simulink model "model"  (R2020b)
settings: Solver=VariableStepAuto  StartTime=0.0  StopTime=1800  RelTol=1e-3
PostLoadFcn:
  | cd(fileparts(which(bdroot)));
  | close all;
  | clear all;
  | clc;
  | set_param('model/switch_v','Label','');
  | set_param('model/switch_h','Label','');
  | set_param('model/switch_T','Label','');
  | set_param('model/switch_P','Label','');
  | set_param('model/switch_m','Label','');
  | set_param('model/switch_p','Label','');
  | set_param('model/switch_slope','Label','');
  | set_param('model/pEtrac','ShowInitialText','off');
  | set_param('model/pErreur+','ShowInitialText','off');
  | set_param('model/pErreur-','ShowInitialText','off');
  | set_param('model/Emodel/Etrac et Erreur/pEtrac','Value','0');
  | set_param('model/Emodel/Etrac et Erreur/pErreur+','Value','0');
  | set_param('model/Emodel/Etrac et Erreur/pErreur-','Value','0');
InitFcn:
  | cd(fileparts(which(bdroot)));
  | load('cycles.mat');
  | clear cycles;
  | cycles = who('-file','cycles.mat');
  | cycleNum = str2num(get_param('model/Emodel/switch_cycles','Value'));
  | cycleName = char(cycles(cycleNum));
  | set_param('model/Emodel/cycle','VariableName',cycleName);
  | cycle = evalin('base',cycleName);
  | T = cycle.time(end);
  | cycleLength = string(T);
  | set_param('model','StopTime',cycleLength);
  | 
  | try
  |  pEtrac = get_param('model/Etrac','Value');
  |  pEtrac = split(pEtrac,'"');
  |  pEtrac = string(pEtrac(2));
  |  set_param('model/Emodel/Etrac et Erreur/pEtrac','Value',pEtrac);
  | 
  |  pErreup = get_param('model/Erreur+','Value');
  |  pErreup = split(pErreup,'"');
  |  pErreup = string(pErreup(2));
  |  set_param('model/Emodel/Etrac et Erreur/pErreur+','Value',pErreup);
  | 
  |  pErreum = get_param('model/Erreur-','Value');
  |  pErreum = split(pErreum,'"');
  |  pErreum = string(pErreum(2));
  |  set_param('model/Emodel/Etrac et Erreur/pErreur-','Value',pErreum);
  | end
StopFcn:
  | sig1Colors.Color = [0 0 1];
  | sig1Colors.LineStyle = '-';
  | sig2Colors.Color = [1 0 0];
  | sig2Colors.LineStyle = '-';
  | sig3Colors.Color = [1 0 0];
  | sig3Colors.LineStyle = '-';
  | sigColors = [sig1Colors sig2Colors sig3Colors];
  | set_param('model/Dashboard_Etrac','Colors',sigColors);
libraries: simulink x1
settings Model: PacingRate=1000  Creator=calexandre  LastModifiedBy=calexandre

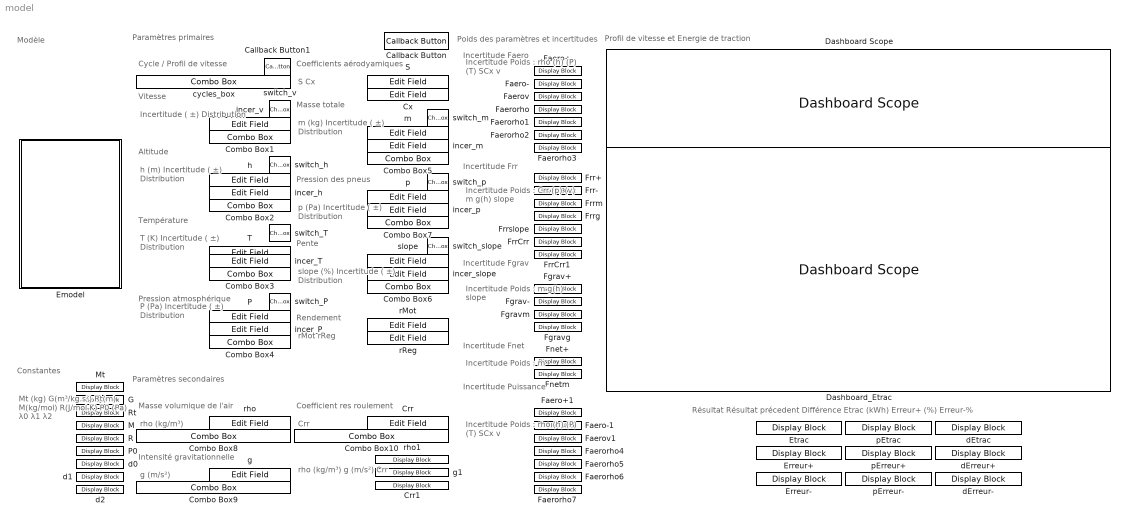
== system model ==
  note: Mt (kg)
      | G(m³/kg.s²)
      | Rt(m)
      | M(kg/mol)
      | R(J/mol.K)
      | P0 (Pa)
      | λ0
      | λ1
      | λ2
  note: Résultat
      | Résultat précedent
      | Différence
      |
      | Etrac (kWh)
      |
      | Erreur+ (%)
      |
      | Erreur-%
  note: Profil de vitesse et Energie de traction
  note: Modèle
  note: Paramètres primaires
  note: Cycle / Profil de vitesse
  note: Incertitude ( ±)
      | Distribution
  note: h (m)
      | Incertitude ( ±)
      | Distribution
  note: Altitude
  note: T (K)
      | Incertitude ( ±)
      | Distribution
  note: Température
  note: P (Pa)
      | Incertitude ( ±)
      | Distribution
  note: Pression atmosphérique
  note: m (kg)
      | Incertitude ( ±)
      | Distribution
  note: Masse totale
  note: slope (%)
      | Incertitude ( ±)
      | Distribution
  note: Pente
  note: p (Pa)
      | Incertitude ( ±)
      | Distribution
  note: Pression des pneus
  note: rho (kg/m³)
  note: Masse volumique de l'air
  note: g (m/s²)
  note: Intensité gravitationnelle
  note: Crr
  note: Coefficient res roulement
  note: S
      | Cx
  note: Coefficients aérodyamiques
  note: Rendement
  note: rMot
      | rReg
  note: Paramètres secondaires
  note: Vitesse
  note: Constantes
  note: Poids des paramètres et incertitudes
  note: rho (kg/m³)
      | g (m/s²)
      | Crr
  note: Incertitude
      | Poids : rho
      | (h)
      | (P)
      | (T)
      | SCx
      | v
  note: Incertitude Faero
  note: Incertitude
      | Poids : Crr
      | (p)
      | (v)
      | m
      | g(h)
      | slope
  note: Incertitude Frr
  note: Incertitude Fgrav
  note: Incertitude
      | Poids : m
      | g(h)
      | slope
  note: Incertitude Fnet
  note: Incertitude
      | Poids : m
  note: Incertitude
      | Poids : rho
      | (h)
      | (P)
      | (T)
      | SCx
      | v
  note: Incertitude Puissance
  Callback Button : CallbackButton  ButtonText=Reset
      settings: ClickFcn=|
      | set_param('model/Emodel/h(m)','Value','0');
      | set_param('model/Emodel/T(K)','Value','285');
      | set_param('model/Emodel/P(Pa)','Value','102900');
      | set_param('model/Emodel/S','Value','2.3');
      | set_param('model/Emodel/Cx','Value','0.36');
      | set_param('model/Emodel/m(kg)','Value','1240');
      | set_param('model/Emodel/p(Pa)','Value','200000');
      | set_param('model/Emodel/slope(%)','Value','0');
      | set_param('model/Emodel/rho(kg.m-3)','Value','1.292');
      | set_param('model/Emodel/g(m.s-2)','Value','9.81');
      | 
      | set_param('model/Emodel/incertitude v','Value','0');
      | set_param('model/Emodel/incertitude h','Value','0');
      | set_param('model/Emodel/incertitude T','Value','0');
      | set_param('model/Emodel/incertitude P','Value','0');
      | set_param('model/Emodel/incertitude m','Value','0');
      | set_param('model/Emodel/incertitude p','Value','0');
      | set_param('model/Emodel/incertitude slope','Value','0');
      | 
      | set_param('model/Emodel/switch incertitude v','Value','0');
      | set_param('model/Emodel/switch incertitude h','Value','0');
      | set_param('model/Emodel/switch incertitude T','Value','0');
      | set_param('model/Emodel/switch incertitude P','Value','0');
      | set_param('model/Emodel/switch incertitude m','Value','0');
      | set_param('model/Emodel/switch incertitude p','Value','0');
      | set_param('model/Emodel/switch incertitude slope','Value','0');
      | 
      | set_param('model/h','FontSize','11');
      | set_param('model/T','FontSize','11');
      | set_param('model/P','FontSize','11');
      | set_param('model/S','FontSize','11');
      | set_param('model/Cx','FontSize','11');
      | set_param('model/m','FontSize','11');
      | set_param('model/p','FontSize','11');
      | set_param('model/slope','FontSize','11');
      | set_param('model/rMot','FontSize','11');
      | set_param('model/rReg','FontSize','11');
      | set_param('model/rho','FontSize','11');
      | set_param('model/g','FontSize','11');
      | set_param('model/Crr','FontSize','11');
      | set_param('model/incer_v','FontSize','11');
      | set_param('model/incer_h','FontSize','11');
      | set_param('model/incer_T','FontSize','11');
      | set_param('model/incer_P','FontSize','11');
      | set_param('model/incer_m','FontSize','11');
      | set_param('model/incer_p','FontSize','11');
      | set_param('model/incer_slope','FontSize','11');
      | set_param('model/Mt','FontSize','11');
      | set_param('model/G','FontSize','11');
      | set_param('model/Rt','FontSize','11');
      | set_param('model/M','FontSize','11');
      | set_param('model/R','FontSize','11');
      | set_param('model/P0','FontSize','11');
      | set_param('model/d0','FontSize','11');
      | set_param('model/d1','FontSize','11');
      | set_param('model/d2','FontSize','11');
      | set_param('model/Etrac','FontSize','11');
      | set_param('model/Erreur+','FontSize','11');
      | set_param('model/Erreur-','FontSize','11');
      | set_param('model/pEtrac','FontSize','11');
      | set_param('model/pErreur+','FontSize','11');
      | set_param('model/pErreur-','FontSize','11');
      | set_param('model/dEtrac','FontSize','11');
      | set_param('model/dErreur+','FontSize','11');
      | set_param('model/dErreur-','FontSize','11');
      | set_param('model/rho1','FontSize','11');
      | set_param('model/g1','FontSize','11');
      | set_param('model/Crr1','FontSize','11');
      | 
      | set_param('model/h','FontSize','12');
      | set_param('model/T','FontSize','12');
      | set_param('model/P','FontSize','12');
      | set_param('model/S','FontSize','12');
      | set_param('model/Cx','FontSize','12');
      | set_param('model/m','FontSize','12');
      | set_param('model/p','FontSize','12');
      | set_param('model/slope','FontSize','12');
      | set_param('model/rMot','FontSize','12');
      | set_param('model/rReg','FontSize','12');
      | set_param('model/rho','FontSize','12');
      | set_param('model/g','FontSize','12');
      | set_param('model/Crr','FontSize','12');
      | set_param('model/incer_v','FontSize','12');
      | set_param('model/incer_h','FontSize','12');
      | set_param('model/incer_T','FontSize','12');
      | set_param('model/incer_P','FontSize','12');
      | set_param('model/incer_m','FontSize','12');
      | set_param('model/incer_p','FontSize','12');
      | set_param('model/incer_slope','FontSize','12');
      | set_param('model/Mt','FontSize','12');
      | set_param('model/G','FontSize','12');
      | set_param('model/Rt','FontSize','12');
      | set_param('model/M','FontSize','12');
      | set_param('model/R','FontSize','12');
      | set_param('model/P0','FontSize','12');
      | set_param('model/d0','FontSize','12');
      | set_param('model/d1','FontSize','12');
      | set_param('model/d2','FontSize','12');
      | set_param('model/Etrac','FontSize','16');
      | set_param('model/Erreur+','FontSize','16');
      | set_param('model/Erreur-','FontSize','16');
      | set_param('model/pEtrac','FontSize','16');
      | set_param('model/pErreur+','FontSize','16');
      | set_param('model/pErreur-','FontSize','16');
      | set_param('model/dEtrac','FontSize','16');
      | set_param('model/dErreur+','FontSize','16');
      | set_param('model/dErreur-','FontSize','16');
      | set_param('model/rho1','FontSize','12');
      | set_param('model/g1','FontSize','12');
      | set_param('model/Crr1','FontSize','12');
  Callback Button1 : CallbackButton  ButtonText=↺
      settings: ClickFcn=|
      | cd(fileparts(which(bdroot)));
      | clear cycles;
      | clear cycles_box_states;
      | cycles = who('-file','cycles.mat');
      | cycles_box_states(length(cycles)) = struct();
      | for i = 1:length(cycles)
      | 	cycles_box_states(i).Value = i;
      |     cycles_box_states(i).Label = char(cycles(i));
      | end
      | set_param('model/cycles_box','States',cycles_box_states);
  Combo Box{1..7} (7 alike) : ComboBox  LabelPosition=Hide  SelectedLabel=Incer-type
      settings: Values={{'Incer-type', 'Gaussienne', 'Rectangulaire', 'Triangle', 'Normale', 'en U'}, [1 2 3 4 5 6]}
  Combo Box10 : ComboBox  LabelPosition=Hide  SelectedLabel=Valeur nominale
      settings: Values={{'Valeur nominale', 'f(p,v)'}, [1 0]}
  Combo Box8 : ComboBox  LabelPosition=Hide  SelectedLabel=Valeur nominale
      settings: Values={{'f(P,T)', 'f(h,T)', 'Valeur nominale'}, [1 2 3]}
  Combo Box9 : ComboBox  LabelPosition=Hide  SelectedLabel=Valeur nominale
      settings: Values={{'Valeur nominale', 'f(h)'}, [0 1]}
  Crr : EditField  LabelPosition=Hide  ShowInitialText=on  Alignment=Center
  Crr1 : DisplayBlock  LabelPosition=Hide  Format=Custom  Transparency=1  FormatString=%.4f
  Cx : EditField  LabelPosition=Hide  ShowInitialText=on  Alignment=Center
  Dashboard Scope : DashboardScope
  Dashboard_Etrac : DashboardScope
  Emodel : Subsystem
  Erreur+ : DisplayBlock  LabelPosition=Hide  Format=short  Transparency=1
  Erreur- : DisplayBlock  LabelPosition=Hide  Format=short  Transparency=1
  Etrac : DisplayBlock  LabelPosition=Hide  Format=short  Transparency=1
  Faero+ : DisplayBlock  LabelPosition=Hide  Format=Custom  Alignment=Right  Transparency=1  FormatString=%.2f N
  Faero+1 : DisplayBlock  LabelPosition=Hide  Format=Custom  Alignment=Right  Transparency=1  FormatString=%.2f N
  Faero- : DisplayBlock  LabelPosition=Hide  Format=Custom  Alignment=Right  Transparency=1  FormatString=%.2f N
  Faero-1 : DisplayBlock  LabelPosition=Hide  Format=Custom  Alignment=Right  Transparency=1  FormatString=%.2f N
  Faerorho{,1..7} (8 alike) : DisplayBlock  LabelPosition=Hide  Format=Custom  Alignment=Right  Transparency=1  FormatString=%.1f %%
  Faerov : DisplayBlock  LabelPosition=Hide  Format=Custom  Alignment=Right  Transparency=1  FormatString=%.1f %%
  Faerov1 : DisplayBlock  LabelPosition=Hide  Format=Custom  Alignment=Right  Transparency=1  FormatString=%.1f %%
  Fgrav+ : DisplayBlock  LabelPosition=Hide  Format=Custom  Alignment=Right  Transparency=1  FormatString=%.2f N
  Fgrav- : DisplayBlock  LabelPosition=Hide  Format=Custom  Alignment=Right  Transparency=1  FormatString=%.2f N
  Fgravg : DisplayBlock  LabelPosition=Hide  Format=Custom  Alignment=Right  Transparency=1  FormatString=%.1f %%
  Fgravm : DisplayBlock  LabelPosition=Hide  Format=Custom  Alignment=Right  Transparency=1  FormatString=%.1f %%
  Fnet+ : DisplayBlock  LabelPosition=Hide  Format=Custom  Alignment=Right  Transparency=1  FormatString=%.2f N
  Fnetm : DisplayBlock  LabelPosition=Hide  Format=Custom  Alignment=Right  Transparency=1  FormatString=%.1f %%
  Frr+ : DisplayBlock  LabelPosition=Hide  Format=Custom  Alignment=Right  Transparency=1  FormatString=%.2f N
  Frr- : DisplayBlock  LabelPosition=Hide  Format=Custom  Alignment=Right  Transparency=1  FormatString=%.2f N
  FrrCrr : DisplayBlock  LabelPosition=Hide  Format=Custom  Alignment=Right  Transparency=1  FormatString=%.1f %%
  FrrCrr1 : DisplayBlock  LabelPosition=Hide  Format=Custom  Alignment=Right  Transparency=1  FormatString=%.1f %%
  Frrg : DisplayBlock  LabelPosition=Hide  Format=Custom  Alignment=Right  Transparency=1  FormatString=%.1f %%
  Frrm : DisplayBlock  LabelPosition=Hide  Format=Custom  Alignment=Right  Transparency=1  FormatString=%.1f %%
  Frrslope : DisplayBlock  LabelPosition=Hide  Format=Custom  Alignment=Right  Transparency=1  FormatString=%.1f %%
  G : DisplayBlock  LabelPosition=Hide  Format=short  Transparency=1
  M : DisplayBlock  LabelPosition=Hide  Format=short  Transparency=1
  Mt : DisplayBlock  LabelPosition=Hide  Format=short  Transparency=1
  P : EditField  LabelPosition=Hide  ShowInitialText=on  Alignment=Center
  P0 : DisplayBlock  LabelPosition=Hide  Format=short  Transparency=1
  R : DisplayBlock  LabelPosition=Hide  Format=short  Transparency=1
  Rt : DisplayBlock  LabelPosition=Hide  Format=short  Transparency=1
  S : EditField  LabelPosition=Hide  ShowInitialText=on  Alignment=Center
  T : EditField  LabelPosition=Hide  ShowInitialText=on  Alignment=Center
  cycles_box : ComboBox  LabelPosition=Hide  SelectedLabel=WLTP_class_3
      settings: Values={{'ArtMw130', 'ArtMw150', 'ArtRoad', 'ArtUrban', 'ECE_R15', 'EUDC', 'FTP', 'HWFET', 'NEDC', 'UDDS', 'WLTP', 'WLTP_class_3'}, [1 2 3 4 5 6 7 8 9 10 11 12]}
  d0 : DisplayBlock  LabelPosition=Hide  Format=short  Transparency=1
  d1 : DisplayBlock  LabelPosition=Hide  Format=short  Transparency=1
  d2 : DisplayBlock  LabelPosition=Hide  Format=short  Transparency=1
  dErreur+ : DisplayBlock  LabelPosition=Hide  ShowInitialText=off  Format=short  Transparency=1
  dErreur- : DisplayBlock  LabelPosition=Hide  ShowInitialText=off  Format=short  Transparency=1
  dEtrac : DisplayBlock  LabelPosition=Hide  ShowInitialText=off  Format=short  Transparency=1
  g : EditField  LabelPosition=Hide  ShowInitialText=on  Alignment=Center
  g1 : DisplayBlock  LabelPosition=Hide  Format=Custom  Transparency=1  FormatString=%.3f m/s²
  h : EditField  LabelPosition=Hide  ShowInitialText=on  Alignment=Center
  incer_P : EditField  LabelPosition=Hide  ShowInitialText=on  Alignment=Center
  incer_T : EditField  LabelPosition=Hide  ShowInitialText=on  Alignment=Center
  incer_h : EditField  LabelPosition=Hide  ShowInitialText=on  Alignment=Center
  incer_m : EditField  LabelPosition=Hide  ShowInitialText=on  Alignment=Center
  incer_p : EditField  LabelPosition=Hide  ShowInitialText=on  Alignment=Center
  incer_slope : EditField  LabelPosition=Hide  ShowInitialText=on  Alignment=Center
  incer_v : EditField  LabelPosition=Hide  ShowInitialText=on  Alignment=Center
  m : EditField  LabelPosition=Hide  ShowInitialText=on  Alignment=Center
  p : EditField  LabelPosition=Hide  ShowInitialText=on  Alignment=Center
  pErreur+ : DisplayBlock  LabelPosition=Hide  ShowInitialText=off  Format=short  Transparency=1
  pErreur- : DisplayBlock  LabelPosition=Hide  ShowInitialText=off  Format=short  Transparency=1
  pEtrac : DisplayBlock  LabelPosition=Hide  ShowInitialText=off  Format=short  Transparency=1
  rMot : EditField  LabelPosition=Hide  ShowInitialText=on  Alignment=Center
  rReg : EditField  LabelPosition=Hide  ShowInitialText=on  Alignment=Center
  rho : EditField  LabelPosition=Hide  ShowInitialText=on  Alignment=Center
  rho1 : DisplayBlock  LabelPosition=Hide  Format=Custom  Transparency=1  FormatString=%.3f kg/m³
  slope : EditField  LabelPosition=Hide  ShowInitialText=on  Alignment=Center
  switch_P : Checkbox  LabelPosition=Hide  ShowInitialText=on
  switch_T : Checkbox  LabelPosition=Hide  ShowInitialText=on
  switch_h : Checkbox  LabelPosition=Hide  ShowInitialText=on
  switch_m : Checkbox  LabelPosition=Hide  ShowInitialText=on
  switch_p : Checkbox  LabelPosition=Hide  ShowInitialText=on
  switch_slope : Checkbox  LabelPosition=Hide  ShowInitialText=on
  switch_v : Checkbox  LabelPosition=Hide  ShowInitialText=on

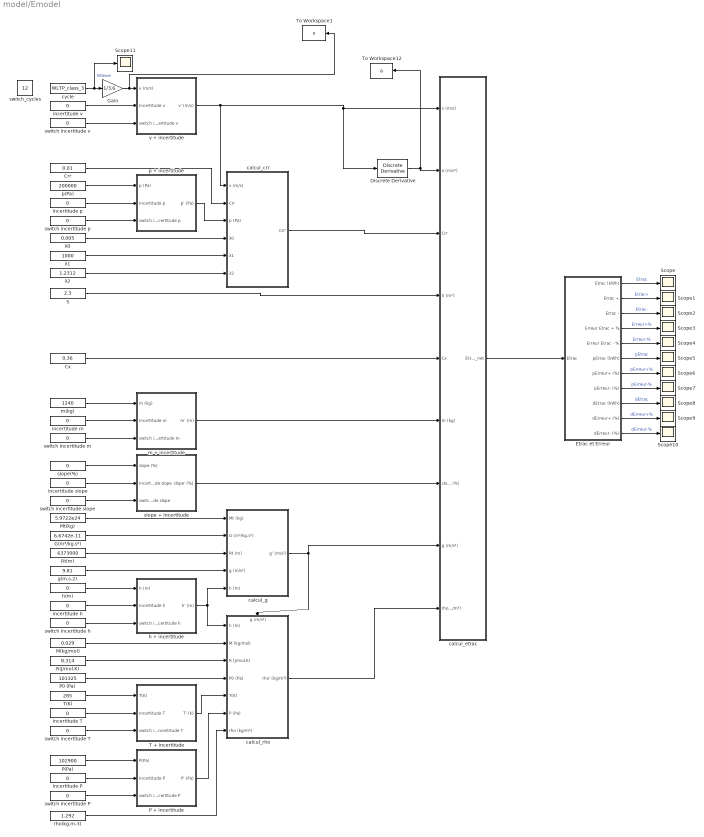
== system model/Emodel ==
  Crr : Constant  Value=0.01
  Cx : Constant  Value=0.36
  Discrete Derivative : simulink/Discrete/Discrete Derivative  gainval=1.0  ICPrevScaledInput=0.0  OutMin=[]  OutMax=[]  OutDataType=fixdt(1, 16)  OutScaling=2^-10  DoSatur=off
  Etrac et Erreur : Subsystem
  G(m³/kg.s²) : Constant  Value=6.6742e-11
  Gain : Gain  Gain=1/3.6
  M(kg/mol) : Constant  Value=0.029
  Mt(kg) : Constant  Value=5.9722e24
  P + incertitude : Subsystem
  P(Pa) : Constant  Value=102900
  P0 (Pa) : Constant  Value=101325
  R(J/mol.K) : Constant  Value=8.314
  Rt(m) : Constant  Value=6373000
  S : Constant  Value=2.3
  Scope{,1..11} (12 alike) : Scope
  T + incertitude : Subsystem
  T(K) : Constant  Value=285
  To Workspace1 : ToWorkspace  VariableName=v  SampleTime=-1
  To Workspace12 : ToWorkspace  VariableName=a  SampleTime=-1
  calcul_crr : Subsystem
  calcul_etrac : Subsystem
  calcul_g : Subsystem
  calcul_rho : Subsystem
      settings: PortSchema="{\"entries\":[{\"content\":{\"sides\":[{\"content\":{\"connectorIds\":[\"In1\",\"In2\",\"In3\",\"In4\",\"In5\",\"In6\",\"In7\"]},\"type\":\"ConnectorPlacement.EquallySpacedRectSide\",\"uuid\":\"cc83d484-c74b-48b3-b83e-1c0f0a113df0\"},{\"content\":{\"connectorIds\":[\"Out1\"],\"side\":\"RIGHT\"},\"type\":\"ConnectorPlacement.EquallySpacedRectSide\",\"uuid\":\"f49ce46b-81e5-420e-b383-21adfa8decb6\"},{\"content\":{\"connectorIds\":[\"In8\"],\"side\":\"TOP\"},\"type\":\"ConnectorPlacement.EquallySpacedRectSide\",\"uuid\":\"3a8f1516-3d8d-4158-a843-5a7993412ec1\"},{\"content\":{\"connectorIds\":[],\"side\":\"HIDDEN\"},\"type\":\"ConnectorPlacement.EquallySpacedRectSide\",\"uuid\":\"5a38b1a2-2dd9-418a-a84f-c8a924db452d\"}]},\"type\":\"ConnectorPlacement.EquallySpacedConnector\",\"uuid\":\"39c01f9e-7b83-41af-a371-ba0a6382fb58\"}],\"packageUris\":[\"http://schema.mathworks.com/mf0/Connector/R2020b\"],\"version\":\"1.0\"}"
  cycle : FromWorkspace  VariableName=WLTP_class_3  SampleTime=1
  g(m.s-2) : Constant  Value=9.81
  h + incertitude : Subsystem
  h(m) : Constant  Value=0
  incertitude P : Constant  Value=0
  incertitude T : Constant  Value=0
  incertitude h : Constant  Value=0
  incertitude m : Constant  Value=0
  incertitude p : Constant  Value=0
  incertitude slope : Constant  Value=0
  incertitude v : Constant  Value=0
  m + incertitude : Subsystem
  m(kg) : Constant  Value=1240
  p + incertitude : Subsystem
  p(Pa) : Constant  Value=200000
  rho(kg.m-3) : Constant  Value=1.292
  slope + incertitude : Subsystem
  slope(%) : Constant  Value=0
  switch incertitude P : Constant  Value=0
  switch incertitude T : Constant  Value=0
  switch incertitude h : Constant  Value=0
  switch incertitude m : Constant  Value=0
  switch incertitude p : Constant  Value=0
  switch incertitude slope : Constant  Value=0
  switch incertitude v : Constant  Value=0
  switch_cycles : Constant  Value=12
  v + incertitude : Subsystem
  λ0 : Constant  Value=0.005
  λ1 : Constant  Value=1000
  λ2 : Constant  Value=1.2312
  wires:
  v + incertitude/1(v' (m/s)) -> calcul_crr/1(v (m/s)), Discrete Derivative/1, calcul_etrac/1(v (m/s))
  Cx/1 -> calcul_etrac/5(Cx)
  S/1 -> calcul_etrac/4(S (m²))
  m + incertitude/1(m' (m)) -> calcul_etrac/6(m (kg))
  M(kg/mol)/1 -> calcul_rho/2(M (kg/mol))
  R(J/mol.K)/1 -> calcul_rho/3(R (J/mol.K))
  calcul_rho/1(rho' (kg/m³)) -> calcul_etrac/9(rho (kg/m³))
  calcul_g/1(g' (m/s²)) -> calcul_rho/8(g (m/s²)), calcul_etrac/8(g (m/s²))
  Mt(kg)/1 -> calcul_g/1(Mt (kg))
  G(m³/kg.s²)/1 -> calcul_g/2(G (m³/kg.s²))
  Rt(m)/1 -> calcul_g/3(Rt (m))
  h + incertitude/1(h' (m)) -> calcul_rho/1(h (m)), calcul_g/5(h (m))
  h(m)/1 -> h + incertitude/1(h (m))
  incertitude h/1 -> h + incertitude/2(Incertitude h)
  switch incertitude h/1 -> h + incertitude/3(switch incertitude h)
  calcul_crr/1(Crr') -> calcul_etrac/3(Crr)
  p(Pa)/1 -> p + incertitude/1(p (Pa))
  p + incertitude/1(p' (Pa)) -> calcul_crr/3(p (Pa))
  incertitude p/1 -> p + incertitude/2(Incertitude p)
  T(K)/1 -> T + incertitude/1(T(K))
  T + incertitude/1(T' (k)) -> calcul_rho/5(T(K))
  switch incertitude T/1 -> T + incertitude/3(switch incertitude T)
  incertitude T/1 -> T + incertitude/2(Incertitude T)
  switch incertitude p/1 -> p + incertitude/3(switch incertitude p)
  switch incertitude slope/1 -> slope + incertitude/3(switch incertitude slope)
  incertitude slope/1 -> slope + incertitude/2(Incertitude slope)
  slope(%)/1 -> slope + incertitude/1(slope (%))
  switch incertitude m/1 -> m + incertitude/3(switch incertitude m)
  incertitude m/1 -> m + incertitude/2(Incertitude m)
  m(kg)/1 -> m + incertitude/1(m (kg))
  slope + incertitude/1(slope' (%)) -> calcul_etrac/7(slope (%))
  Gain/1 -> To Workspace1/1, v + incertitude/1(v (m/s))
  incertitude v/1 -> v + incertitude/2(Incertitude v)
  switch incertitude v/1 -> v + incertitude/3(switch incertitude v)
  P(Pa)/1 -> P + incertitude/1(P(Pa))
  incertitude P/1 -> P + incertitude/2(Incertitude P)
  switch incertitude P/1 -> P + incertitude/3(switch incertitude P)
  P + incertitude/1(P' (Pa)) -> calcul_rho/6(P (Pa))
  rho(kg.m-3)/1 -> calcul_rho/7(rho (kg/m³))
  g(m.s-2)/1 -> calcul_g/4(g (m/s²))
  Crr/1 -> calcul_crr/2(Crr)
  calcul_etrac/1(Etraction_net) -> Etrac et Erreur/1(Etrac)
  Etrac et Erreur/2(Etrac +) -> Scope1/1  "Etrac+"
  Etrac et Erreur/3(Etrac -) -> Scope2/1  "Etrac-"
  Discrete Derivative/1 -> To Workspace12/1, calcul_etrac/2(a (m/s²))
  Etrac et Erreur/4(Erreur Etrac + %) -> Scope3/1  "Erreur+%"
  Etrac et Erreur/1(Etrac (kWh)) -> Scope/1  "Etrac"
  Etrac et Erreur/5(Erreur Etrac - %) -> Scope4/1  "Erreur-%"
  Etrac et Erreur/6(pEtrac (kWh)) -> Scope5/1  "pEtrac"
  Etrac et Erreur/7(pErreur+ (%)) -> Scope6/1  "pErreur+%"
  Etrac et Erreur/8(pErreur- (%)) -> Scope7/1  "pErreur-%"
  Etrac et Erreur/9(dEtrac (kWh)) -> Scope8/1  "dEtrac"
  Etrac et Erreur/10(dErreur+ (%)) -> Scope9/1  "dErreur+%"
  Etrac et Erreur/11(dErreur- (%)) -> Scope10/1  "dErreur-%"
  P0 (Pa)/1 -> calcul_rho/4(P0 (Pa))
  λ0/1 -> calcul_crr/4(λ0)
  λ1/1 -> calcul_crr/5(λ1)
  λ2/1 -> calcul_crr/6(λ2)
  cycle/1 -> Scope11/1, Gain/1  "Vitesse"

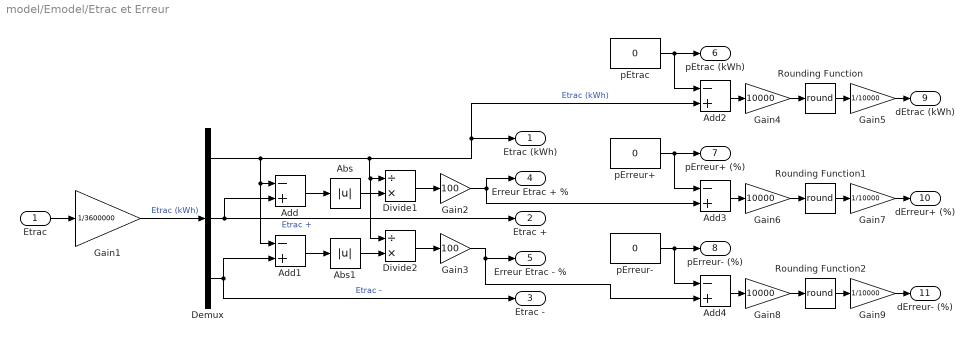
== system model/Emodel/Etrac et Erreur ==
  Etrac : Inport
  Abs : Abs
  Abs1 : Abs
  Add{,1..4} (5 alike) : Sum  Inputs=-+
  Demux : Demux  Outputs=3
  Divide1 : Product  Inputs=/*
  Divide2 : Product  Inputs=/*
  Gain1 : Gain  Gain=1/3600000
  Gain2 : Gain  Gain=100
  Gain3 : Gain  Gain=100
  Gain4 : Gain  Gain=10000
  Gain5 : Gain  Gain=1/10000
  Gain6 : Gain  Gain=10000
  Gain7 : Gain  Gain=1/10000
  Gain8 : Gain  Gain=10000
  Gain9 : Gain  Gain=1/10000
  Rounding Function : Rounding  Operator=round
  Rounding Function1 : Rounding  Operator=round
  Rounding Function2 : Rounding  Operator=round
  pErreur+ : Constant  Value=0
  pErreur- : Constant  Value=0
  pEtrac : Constant  Value=0
  Etrac (kWh) : Outport
  Etrac + : Outport  Port=2
  Etrac - : Outport  Port=3
  Erreur Etrac + % : Outport  Port=4
  Erreur Etrac - % : Outport  Port=5
  pEtrac (kWh) : Outport  Port=6
  pErreur+ (%) : Outport  Port=7
  pErreur- (%) : Outport  Port=8
  dEtrac (kWh) : Outport  Port=9
  dErreur+ (%) : Outport  Port=10
  dErreur- (%) : Outport  Port=11
  wires:
  Divide1/1 -> Gain2/1
  Add/1 -> Abs/1
  Demux/2 -> Etrac +/1, Add/2  "Etrac +"
  Demux/1 -> Add2/2, Etrac (kWh)/1, Divide2/1, Divide1/1, Add1/1, Add/1  "Etrac (kWh)"
  Gain1/1 -> Demux/1  "Etrac (kWh)"
  Etrac/1 -> Gain1/1
  Abs/1 -> Divide1/2
  Demux/3 -> Add1/2, Etrac -/1  "Etrac -"
  Gain2/1 -> Add3/2, Erreur Etrac + %/1
  Add1/1 -> Abs1/1
  Divide2/1 -> Gain3/1
  Gain3/1 -> Add4/2, Erreur Etrac - %/1
  Abs1/1 -> Divide2/2
  Rounding Function/1 -> Gain5/1
  Gain4/1 -> Rounding Function/1
  pEtrac/1 -> pEtrac (kWh)/1, Add2/1
  Gain5/1 -> dEtrac (kWh)/1
  Add2/1 -> Gain4/1
  Gain7/1 -> dErreur+ (%)/1
  Add3/1 -> Gain6/1
  pErreur+/1 -> pErreur+ (%)/1, Add3/1
  Gain6/1 -> Rounding Function1/1
  Rounding Function1/1 -> Gain7/1
  Gain9/1 -> dErreur- (%)/1
  Add4/1 -> Gain8/1
  pErreur-/1 -> pErreur- (%)/1, Add4/1
  Gain8/1 -> Rounding Function2/1
  Rounding Function2/1 -> Gain9/1

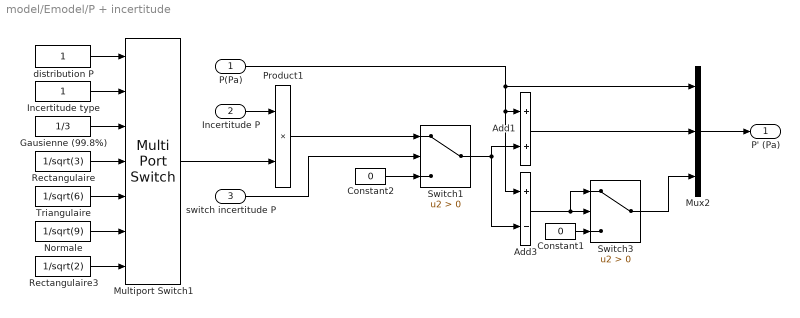
== system model/Emodel/P + incertitude ==
  P(Pa) : Inport
  Incertitude P : Inport  Port=2
  switch incertitude P : Inport  Port=3
  Add1 : Sum
  Add3 : Sum  Inputs=+-
  Constant1 : Constant  Value=0
  Constant2 : Constant  Value=0
  Gausienne (99.8%) : Constant  Value=1/3
  Incertitude type : Constant
  Multiport Switch1 : MultiPortSwitch  Inputs=6
  Mux2 : Mux  Inputs=3
  Normale : Constant  Value=1/sqrt(9)
  Product1 : Product
  Rectangulaire : Constant  Value=1/sqrt(3)
  Rectangulaire3 : Constant  Value=1/sqrt(2)
  Switch1 : Switch  Criteria=u2 > Threshold
  Switch3 : Switch  Criteria=u2 > Threshold
  Triangulaire : Constant  Value=1/sqrt(6)
  distribution P : Constant
  P' (Pa) : Outport
  wires:
  Normale/1 -> Multiport Switch1/6
  Rectangulaire3/1 -> Multiport Switch1/7
  Rectangulaire/1 -> Multiport Switch1/4
  Multiport Switch1/1 -> Product1/2
  Incertitude type/1 -> Multiport Switch1/2
  Triangulaire/1 -> Multiport Switch1/5
  Gausienne (99.8%)/1 -> Multiport Switch1/3
  distribution P/1 -> Multiport Switch1/1
  Incertitude P/1 -> Product1/1
  Mux2/1 -> P' (Pa)/1
  Switch1/1 -> Add3/2, Add1/2
  Product1/1 -> Switch1/1
  Constant2/1 -> Switch1/3
  switch incertitude P/1 -> Switch1/2
  P(Pa)/1 -> Add3/1, Add1/1, Mux2/1
  Constant1/1 -> Switch3/3
  Add3/1 -> Switch3/1, Switch3/2
  Add1/1 -> Mux2/2
  Switch3/1 -> Mux2/3

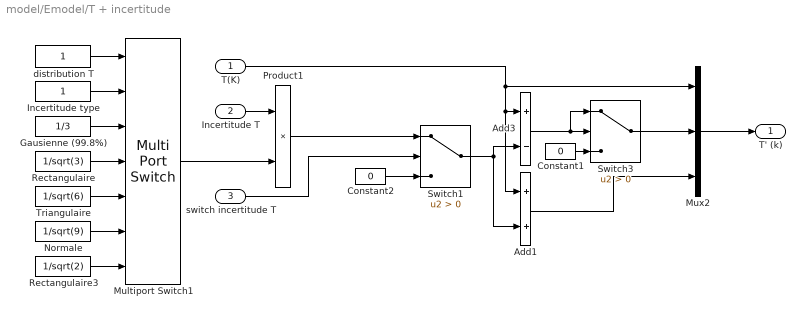
== system model/Emodel/T + incertitude ==
  T(K) : Inport
  Incertitude T : Inport  Port=2
  switch incertitude T : Inport  Port=3
  Add1 : Sum
  Add3 : Sum  Inputs=+-
  Constant1 : Constant  Value=0
  Constant2 : Constant  Value=0
  Gausienne (99.8%) : Constant  Value=1/3
  Incertitude type : Constant
  Multiport Switch1 : MultiPortSwitch  Inputs=6
  Mux2 : Mux  Inputs=3
  Normale : Constant  Value=1/sqrt(9)
  Product1 : Product
  Rectangulaire : Constant  Value=1/sqrt(3)
  Rectangulaire3 : Constant  Value=1/sqrt(2)
  Switch1 : Switch  Criteria=u2 > Threshold
  Switch3 : Switch  Criteria=u2 > Threshold
  Triangulaire : Constant  Value=1/sqrt(6)
  distribution T : Constant
  T' (k) : Outport
  wires:
  Normale/1 -> Multiport Switch1/6
  Rectangulaire3/1 -> Multiport Switch1/7
  Product1/1 -> Switch1/1
  Rectangulaire/1 -> Multiport Switch1/4
  Multiport Switch1/1 -> Product1/2
  Incertitude type/1 -> Multiport Switch1/2
  Triangulaire/1 -> Multiport Switch1/5
  Gausienne (99.8%)/1 -> Multiport Switch1/3
  distribution T/1 -> Multiport Switch1/1
  switch incertitude T/1 -> Switch1/2
  Mux2/1 -> T' (k)/1
  Incertitude T/1 -> Product1/1
  Constant2/1 -> Switch1/3
  Add3/1 -> Switch3/1, Switch3/2
  T(K)/1 -> Add1/1, Add3/1, Mux2/1
  Constant1/1 -> Switch3/3
  Switch1/1 -> Add1/2, Add3/2
  Switch3/1 -> Mux2/2
  Add1/1 -> Mux2/3

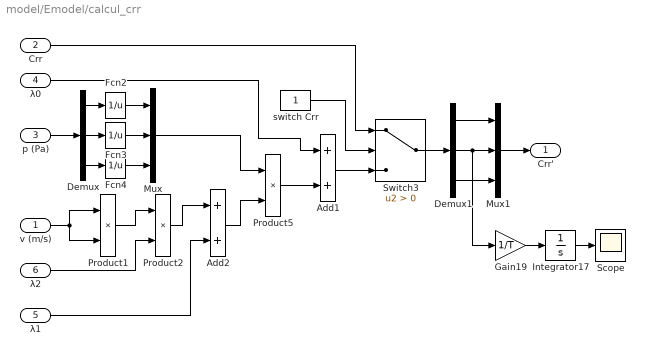
== system model/Emodel/calcul_crr ==
  v (m/s) : Inport
  Crr : Inport  Port=2
  p (Pa) : Inport  Port=3
  λ0 : Inport  Port=4
  λ1 : Inport  Port=5
  λ2 : Inport  Port=6
  Add1 : Sum
  Add2 : Sum
  Demux : Demux  Outputs=3
  Demux1 : Demux  Outputs=3
  Fcn2 : Fcn  Expr=1/u
  Fcn3 : Fcn  Expr=1/u
  Fcn4 : Fcn  Expr=1/u
  Gain19 : Gain  Gain=1/T
  Integrator17 : Integrator
  Mux : Mux  Inputs=3
  Mux1 : Mux  Inputs=3
  Product1 : Product
  Product2 : Product
  Product5 : Product
  Scope : Scope
  Switch3 : Switch  Criteria=u2 > Threshold
  switch Crr : Constant
  Crr' : Outport
  wires:
  Product5/1 -> Add1/2
  switch Crr/1 -> Switch3/2
  λ0/1 -> Add1/1
  Add1/1 -> Switch3/3
  Crr/1 -> Switch3/1
  Switch3/1 -> Demux1/1
  p (Pa)/1 -> Demux/1
  Demux/1 -> Fcn2/1
  Demux/2 -> Fcn3/1
  Demux/3 -> Fcn4/1
  Fcn2/1 -> Mux/1
  Fcn3/1 -> Mux/2
  Fcn4/1 -> Mux/3
  Mux/1 -> Product5/1
  v (m/s)/1 -> Product1/1, Product1/2
  Product1/1 -> Product2/1
  Add2/1 -> Product5/2
  Product2/1 -> Add2/1
  λ2/1 -> Product2/2
  λ1/1 -> Add2/2
  Demux1/3 -> Mux1/3
  Demux1/1 -> Mux1/1
  Demux1/2 -> Gain19/1, Mux1/2
  Mux1/1 -> Crr'/1
  Gain19/1 -> Integrator17/1
  Integrator17/1 -> Scope/1

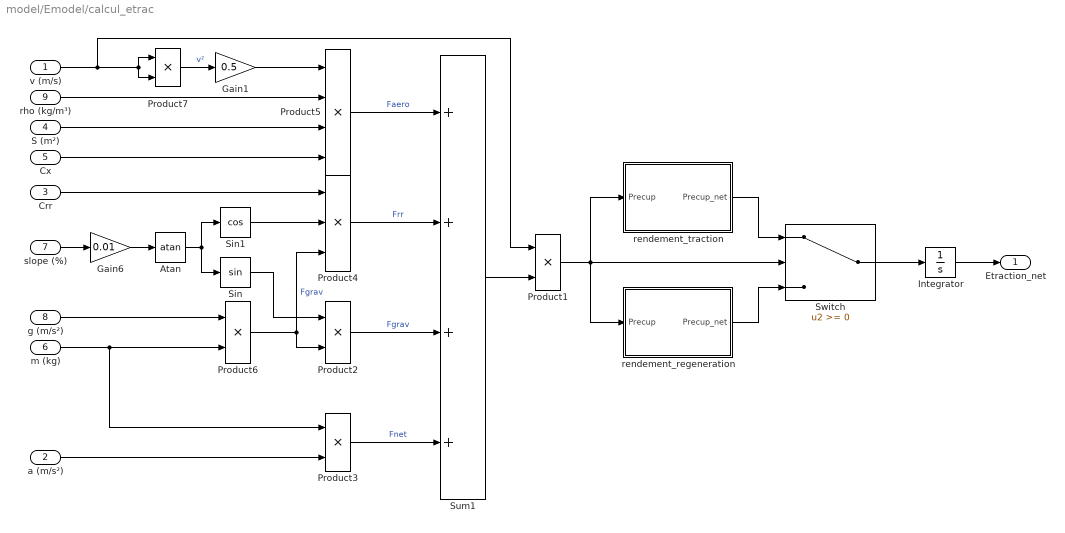
== system model/Emodel/calcul_etrac ==
  v (m/s) : Inport
  a (m/s²) : Inport  Port=2
  Crr : Inport  Port=3
  S (m²) : Inport  Port=4
  Cx : Inport  Port=5
  m (kg) : Inport  Port=6
  slope (%) : Inport  Port=7
  g (m/s²) : Inport  Port=8
  rho (kg/m³) : Inport  Port=9
  Atan : Trigonometry  Operator=atan
  Gain1 : Gain  Gain=0.5
  Gain6 : Gain  Gain=0.01
  Integrator : Integrator
  Product{1..3,6..7} (5 alike) : Product
  Product4 : Product  Inputs=3
  Product5 : Product  Inputs=4
  Sin : Trigonometry
  Sin1 : Trigonometry  Operator=cos
  Sum1 : Sum  Inputs=++++
  Switch : Switch
  rendement_regeneration : Subsystem
  rendement_traction : Subsystem
  Etraction_net : Outport  VectorParamsAs1DForOutWhenUnconnected=off
  wires:
  Switch/1 -> Integrator/1
  Sum1/1 -> Product1/2
  Product4/1 -> Sum1/2  "Frr"
  slope (%)/1 -> Gain6/1
  Product3/1 -> Sum1/4  "Fnet"
  Product7/1 -> Gain1/1  "v²"
  a (m/s²)/1 -> Product3/2
  Product5/1 -> Sum1/1  "Faero"
  v (m/s)/1 -> Product7/1, Product7/2, Product1/1
  Integrator/1 -> Etraction_net/1
  Product1/1 -> rendement_regeneration/1(Precup), rendement_traction/1(Precup), Switch/2
  g (m/s²)/1 -> Product6/1
  Gain6/1 -> Atan/1
  m (kg)/1 -> Product6/2, Product3/1
  S (m²)/1 -> Product5/3
  rho (kg/m³)/1 -> Product5/2
  Cx/1 -> Product5/4
  Gain1/1 -> Product5/1
  Crr/1 -> Product4/1
  Product2/1 -> Sum1/3  "Fgrav"
  Sin1/1 -> Product4/2
  Product6/1 -> Product2/2, Product4/3  "Fgrav"
  Sin/1 -> Product2/1
  rendement_regeneration/1(Precup_net) -> Switch/3
  rendement_traction/1(Precup_net) -> Switch/1
  Atan/1 -> Sin/1, Sin1/1

== system model/Emodel/calcul_g ==
  Mt (kg) : Inport
  G (m³/kg.s²) : Inport  Port=2
  Rt (m) : Inport  Port=3
  g (m/s²) : Inport  Port=4
  h (m) : Inport  Port=5
  Add : Sum
  Demux1 : Demux  Outputs=3
  Divide : Product  Inputs=*/
  Gain19 : Gain  Gain=1/T
  Integrator17 : Integrator
  Mux1 : Mux  Inputs=3
  Product : Product
  Product1 : Product
  Scope : Scope
  Switch : Switch  Criteria=u2 > Threshold
  switch g : Constant  Value=0
  g' (m/s²) : Outport
  wires:
  Product1/1 -> Divide/2
  Product/1 -> Divide/1
  Divide/1 -> Switch/1
  g (m/s²)/1 -> Switch/3
  switch g/1 -> Switch/2
  h (m)/1 -> Add/2
  Add/1 -> Product1/1, Product1/2
  G (m³/kg.s²)/1 -> Product/2
  Mt (kg)/1 -> Product/1
  Rt (m)/1 -> Add/1
  Mux1/1 -> g' (m/s²)/1
  Switch/1 -> Demux1/1
  Demux1/3 -> Mux1/3
  Demux1/1 -> Mux1/1
  Gain19/1 -> Integrator17/1
  Demux1/2 -> Gain19/1, Mux1/2
  Integrator17/1 -> Scope/1

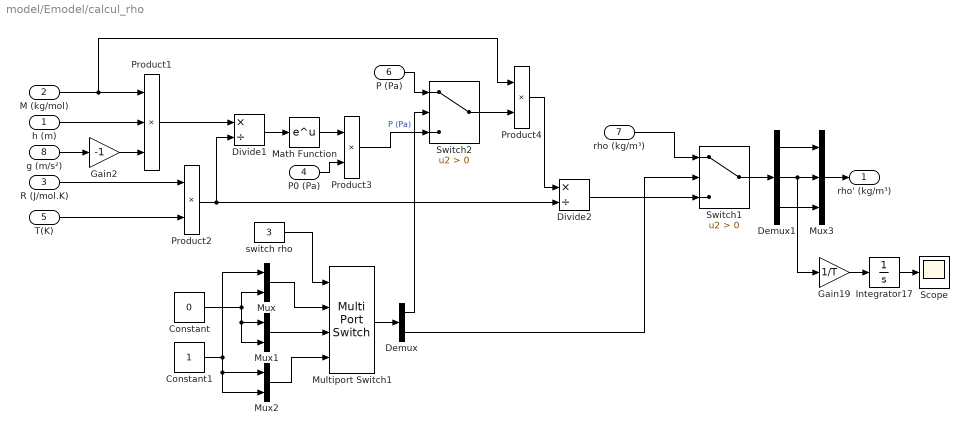
== system model/Emodel/calcul_rho ==
  h (m) : Inport
  M (kg/mol) : Inport  Port=2
  R (J/mol.K) : Inport  Port=3
  P0 (Pa) : Inport  Port=4
  T(K) : Inport  Port=5
  P (Pa) : Inport  Port=6
  rho (kg/m³) : Inport  Port=7
  g (m/s²) : Inport  Port=8
  Constant : Constant  Value=0
  Constant1 : Constant
  Demux : Demux  Outputs=2
  Demux1 : Demux  Outputs=3
  Divide1 : Product  Inputs=*/
  Divide2 : Product  Inputs=*/
  Gain19 : Gain  Gain=1/T
  Gain2 : Gain  Gain=-1
  Integrator17 : Integrator
  Math Function : Math  SaturateOnIntegerOverflow=on
  Multiport Switch1 : MultiPortSwitch
  Mux : Mux  Inputs=2
  Mux1 : Mux  Inputs=2
  Mux2 : Mux  Inputs=2
  Mux3 : Mux  Inputs=3
  Product1 : Product  Inputs=3
  Product2 : Product
  Product3 : Product
  Product4 : Product
  Scope : Scope
  Switch1 : Switch  Criteria=u2 > Threshold
  Switch2 : Switch  Criteria=u2 > Threshold
  switch rho : Constant  Value=3
  rho' (kg/m³) : Outport
  wires:
  Divide1/1 -> Math Function/1
  Product2/1 -> Divide1/2, Divide2/2
  Product4/1 -> Divide2/1
  Switch2/1 -> Product4/2
  Product3/1 -> Switch2/3  "P (Pa)"
  Math Function/1 -> Product3/1
  P (Pa)/1 -> Switch2/1
  rho (kg/m³)/1 -> Switch1/1
  Divide2/1 -> Switch1/3
  R (J/mol.K)/1 -> Product2/1
  g (m/s²)/1 -> Gain2/1
  h (m)/1 -> Product1/2
  T(K)/1 -> Product2/2
  M (kg/mol)/1 -> Product1/1, Product4/1
  Gain2/1 -> Product1/3
  P0 (Pa)/1 -> Product3/2
  switch rho/1 -> Multiport Switch1/1
  Multiport Switch1/1 -> Demux/1
  Demux/1 -> Switch2/2
  Demux/2 -> Switch1/2
  Mux/1 -> Multiport Switch1/2
  Mux1/1 -> Multiport Switch1/3
  Mux2/1 -> Multiport Switch1/4
  Constant1/1 -> Mux2/2, Mux2/1, Mux/1
  Constant/1 -> Mux/2, Mux1/1, Mux1/2
  Product1/1 -> Divide1/1
  Mux3/1 -> rho' (kg/m³)/1
  Switch1/1 -> Demux1/1
  Demux1/3 -> Mux3/3
  Demux1/1 -> Mux3/1
  Gain19/1 -> Integrator17/1
  Demux1/2 -> Gain19/1, Mux3/2
  Integrator17/1 -> Scope/1

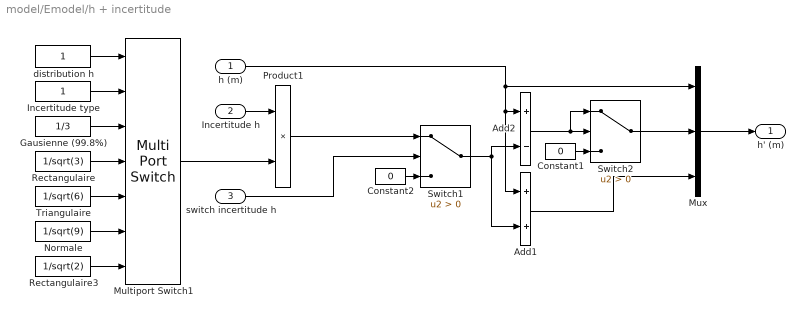
== system model/Emodel/h + incertitude ==
  h (m) : Inport
  Incertitude h : Inport  Port=2
  switch incertitude h : Inport  Port=3
  Add1 : Sum
  Add2 : Sum  Inputs=+-
  Constant1 : Constant  Value=0
  Constant2 : Constant  Value=0
  Gausienne (99.8%) : Constant  Value=1/3
  Incertitude type : Constant
  Multiport Switch1 : MultiPortSwitch  Inputs=6
  Mux : Mux  Inputs=3
  Normale : Constant  Value=1/sqrt(9)
  Product1 : Product
  Rectangulaire : Constant  Value=1/sqrt(3)
  Rectangulaire3 : Constant  Value=1/sqrt(2)
  Switch1 : Switch  Criteria=u2 > Threshold
  Switch2 : Switch  Criteria=u2 > Threshold
  Triangulaire : Constant  Value=1/sqrt(6)
  distribution h : Constant
  h' (m) : Outport
  wires:
  Normale/1 -> Multiport Switch1/6
  Rectangulaire3/1 -> Multiport Switch1/7
  Product1/1 -> Switch1/1
  Rectangulaire/1 -> Multiport Switch1/4
  Multiport Switch1/1 -> Product1/2
  Incertitude type/1 -> Multiport Switch1/2
  Triangulaire/1 -> Multiport Switch1/5
  Gausienne (99.8%)/1 -> Multiport Switch1/3
  distribution h/1 -> Multiport Switch1/1
  switch incertitude h/1 -> Switch1/2
  Mux/1 -> h' (m)/1
  Incertitude h/1 -> Product1/1
  Constant2/1 -> Switch1/3
  h (m)/1 -> Add1/1, Add2/1, Mux/1
  Switch1/1 -> Add1/2, Add2/2
  Add2/1 -> Switch2/1, Switch2/2
  Constant1/1 -> Switch2/3
  Switch2/1 -> Mux/2
  Add1/1 -> Mux/3

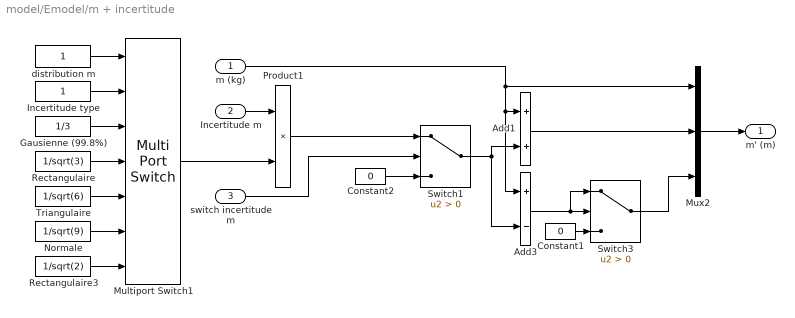
== system model/Emodel/m + incertitude ==
  m (kg) : Inport
  Incertitude m : Inport  Port=2
  switch incertitude m : Inport  Port=3
  Add1 : Sum
  Add3 : Sum  Inputs=+-
  Constant1 : Constant  Value=0
  Constant2 : Constant  Value=0
  Gausienne (99.8%) : Constant  Value=1/3
  Incertitude type : Constant
  Multiport Switch1 : MultiPortSwitch  Inputs=6
  Mux2 : Mux  Inputs=3
  Normale : Constant  Value=1/sqrt(9)
  Product1 : Product
  Rectangulaire : Constant  Value=1/sqrt(3)
  Rectangulaire3 : Constant  Value=1/sqrt(2)
  Switch1 : Switch  Criteria=u2 > Threshold
  Switch3 : Switch  Criteria=u2 > Threshold
  Triangulaire : Constant  Value=1/sqrt(6)
  distribution m : Constant
  m' (m) : Outport
  wires:
  Normale/1 -> Multiport Switch1/6
  Rectangulaire3/1 -> Multiport Switch1/7
  Rectangulaire/1 -> Multiport Switch1/4
  Multiport Switch1/1 -> Product1/2
  Incertitude type/1 -> Multiport Switch1/2
  Triangulaire/1 -> Multiport Switch1/5
  Gausienne (99.8%)/1 -> Multiport Switch1/3
  distribution m/1 -> Multiport Switch1/1
  Incertitude m/1 -> Product1/1
  Product1/1 -> Switch1/1
  Add1/1 -> Mux2/2
  Constant1/1 -> Switch3/3
  Add3/1 -> Switch3/1, Switch3/2
  Switch3/1 -> Mux2/3
  Constant2/1 -> Switch1/3
  Mux2/1 -> m' (m)/1
  m (kg)/1 -> Add3/1, Add1/1, Mux2/1
  Switch1/1 -> Add3/2, Add1/2
  switch incertitude m/1 -> Switch1/2

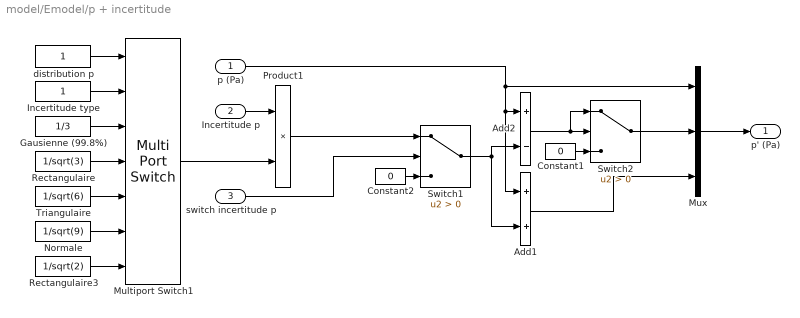
== system model/Emodel/p + incertitude ==
  p (Pa) : Inport
  Incertitude p : Inport  Port=2
  switch incertitude p : Inport  Port=3
  Add1 : Sum
  Add2 : Sum  Inputs=+-
  Constant1 : Constant  Value=0
  Constant2 : Constant  Value=0
  Gausienne (99.8%) : Constant  Value=1/3
  Incertitude type : Constant
  Multiport Switch1 : MultiPortSwitch  Inputs=6
  Mux : Mux  Inputs=3
  Normale : Constant  Value=1/sqrt(9)
  Product1 : Product
  Rectangulaire : Constant  Value=1/sqrt(3)
  Rectangulaire3 : Constant  Value=1/sqrt(2)
  Switch1 : Switch  Criteria=u2 > Threshold
  Switch2 : Switch  Criteria=u2 > Threshold
  Triangulaire : Constant  Value=1/sqrt(6)
  distribution p : Constant
  p' (Pa) : Outport
  wires:
  Normale/1 -> Multiport Switch1/6
  Rectangulaire3/1 -> Multiport Switch1/7
  Rectangulaire/1 -> Multiport Switch1/4
  Multiport Switch1/1 -> Product1/2
  Incertitude type/1 -> Multiport Switch1/2
  Triangulaire/1 -> Multiport Switch1/5
  Gausienne (99.8%)/1 -> Multiport Switch1/3
  distribution p/1 -> Multiport Switch1/1
  Incertitude p/1 -> Product1/1
  Add2/1 -> Switch2/1, Switch2/2
  p (Pa)/1 -> Add1/1, Add2/1, Mux/1
  Constant1/1 -> Switch2/3
  Switch2/1 -> Mux/2
  Add1/1 -> Mux/3
  Switch1/1 -> Add1/2, Add2/2
  Constant2/1 -> Switch1/3
  switch incertitude p/1 -> Switch1/2
  Mux/1 -> p' (Pa)/1
  Product1/1 -> Switch1/1

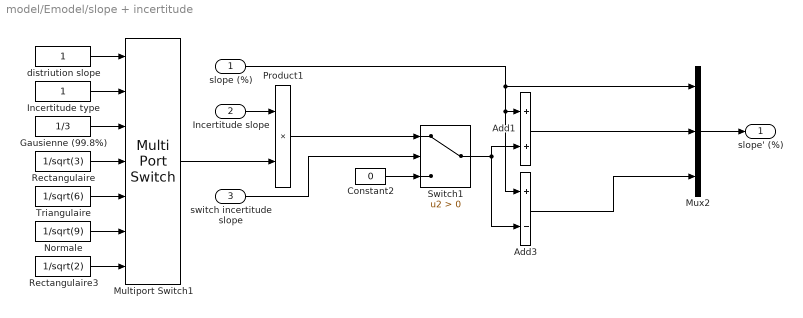
== system model/Emodel/slope + incertitude ==
  slope (%) : Inport
  Incertitude slope : Inport  Port=2
  switch incertitude slope : Inport  Port=3
  Add1 : Sum
  Add3 : Sum  Inputs=+-
  Constant2 : Constant  Value=0
  Gausienne (99.8%) : Constant  Value=1/3
  Incertitude type : Constant
  Multiport Switch1 : MultiPortSwitch  Inputs=6
  Mux2 : Mux  Inputs=3
  Normale : Constant  Value=1/sqrt(9)
  Product1 : Product
  Rectangulaire : Constant  Value=1/sqrt(3)
  Rectangulaire3 : Constant  Value=1/sqrt(2)
  Switch1 : Switch  Criteria=u2 > Threshold
  Triangulaire : Constant  Value=1/sqrt(6)
  distriution slope : Constant
  slope' (%) : Outport
  wires:
  Normale/1 -> Multiport Switch1/6
  Rectangulaire3/1 -> Multiport Switch1/7
  Rectangulaire/1 -> Multiport Switch1/4
  Multiport Switch1/1 -> Product1/2
  Incertitude type/1 -> Multiport Switch1/2
  Triangulaire/1 -> Multiport Switch1/5
  Gausienne (99.8%)/1 -> Multiport Switch1/3
  distriution slope/1 -> Multiport Switch1/1
  Incertitude slope/1 -> Product1/1
  Product1/1 -> Switch1/1
  Add1/1 -> Mux2/2
  Constant2/1 -> Switch1/3
  Mux2/1 -> slope' (%)/1
  slope (%)/1 -> Add3/1, Add1/1, Mux2/1
  Switch1/1 -> Add3/2, Add1/2
  switch incertitude slope/1 -> Switch1/2
  Add3/1 -> Mux2/3

== system model/Emodel/v + incertitude ==
  v (m/s) : Inport
  Incertitude v : Inport  Port=2
  switch incertitude v : Inport  Port=3
  Add1 : Sum
  Add3 : Sum  Inputs=+-
  Constant2 : Constant  Value=0
  Gausienne (99.8%) : Constant  Value=1/3
  Incertitude type : Constant
  Multiport Switch1 : MultiPortSwitch  Inputs=6
  Mux2 : Mux  Inputs=3
  Normale : Constant  Value=1/sqrt(9)
  Product1 : Product
  Rectangulaire : Constant  Value=1/sqrt(3)
  Rectangulaire3 : Constant  Value=1/sqrt(2)
  Switch1 : Switch  Criteria=u2 > Threshold
  Triangulaire : Constant  Value=1/sqrt(6)
  distribution v : Constant
  v' (m/s) : Outport
  wires:
  Normale/1 -> Multiport Switch1/6
  Rectangulaire3/1 -> Multiport Switch1/7
  Rectangulaire/1 -> Multiport Switch1/4
  Multiport Switch1/1 -> Product1/2
  Incertitude type/1 -> Multiport Switch1/2
  Triangulaire/1 -> Multiport Switch1/5
  Gausienne (99.8%)/1 -> Multiport Switch1/3
  distribution v/1 -> Multiport Switch1/1
  Incertitude v/1 -> Product1/1
  Constant2/1 -> Switch1/3
  Switch1/1 -> Add3/2, Add1/2
  Add1/1 -> Mux2/2
  Product1/1 -> Switch1/1
  switch incertitude v/1 -> Switch1/2
  v (m/s)/1 -> Add3/1, Add1/1, Mux2/1
  Mux2/1 -> v' (m/s)/1
  Add3/1 -> Mux2/3

== system model/Emodel/calcul_etrac/rendement_regeneration ==
  Precup : Inport
  rendement : Gain  Gain=0.6774
  Precup_net : Outport  VectorParamsAs1DForOutWhenUnconnected=off
  wires:
  Precup/1 -> rendement/1
  rendement/1 -> Precup_net/1

== system model/Emodel/calcul_etrac/rendement_traction ==
  Precup : Inport
  rendement : Gain  Gain=1/ 0.8216
  Precup_net : Outport  VectorParamsAs1DForOutWhenUnconnected=off
  wires:
  Precup/1 -> rendement/1
  rendement/1 -> Precup_net/1
